simulink model "FrequencyResponseTester"  (R2023b)
settings: Solver=VariableStepAuto  StartTime=0.0  StopTime=10.0  RelTol=1e-3
libraries: simulink x1, c2838x_M4_lib x1
settings Model: Creator=Administrator  LastModifiedBy=Administrator

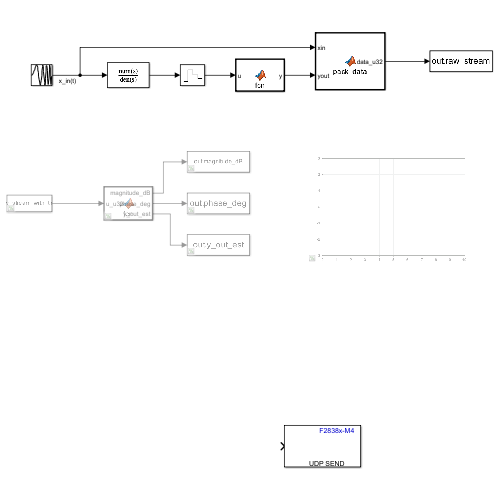
[thumbnail: Simulink's stored preview of the top-level diagram]
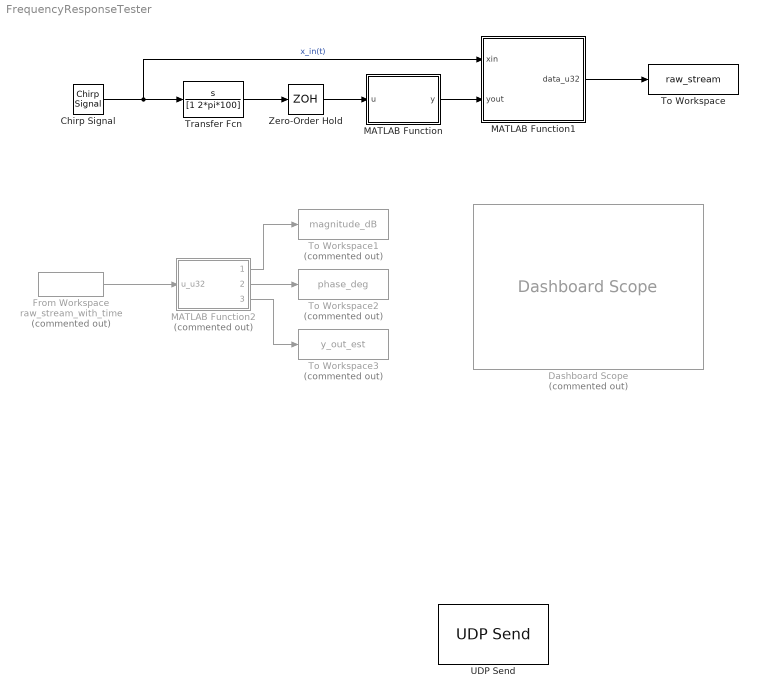
== system FrequencyResponseTester ==
  Chirp Signal : simulink/Sources/Chirp Signal  f1=1  T=10  f2=1000
  Dashboard Scope : DashboardScope  Commented=on
  From Workspace : FromWorkspace  Commented=on  VariableName=raw_stream_with_time  SampleTime=1e-4  OutputAfterFinalValue=Holding final value
  MATLAB Function : MATLAB Function  TreatAsAtomicUnit=on
  MATLAB Function1 : MATLAB Function  TreatAsAtomicUnit=on
  MATLAB Function2 : MATLAB Function  Commented=on  TreatAsAtomicUnit=on
  To Workspace : ToWorkspace  VariableName=raw_stream  SaveFormat=Timeseries  SampleTime=1e-4
  To Workspace1 : ToWorkspace  Commented=on  VariableName=magnitude_dB  SaveFormat=Timeseries  SampleTime=-1
  To Workspace2 : ToWorkspace  Commented=on  VariableName=phase_deg  SaveFormat=Timeseries  SampleTime=-1
  To Workspace3 : ToWorkspace  Commented=on  VariableName=y_out_est  SaveFormat=Timeseries  SampleTime=-1
  Transfer Fcn : TransferFcn  Numerator=[1 0]  Denominator=[1 2*pi*100]
  UDP Send : c2838x_M4_lib/UDP Send  RemoteIPAddress_=127.0.0.1  RemoteIPPort_=25000  LocalIPPort_=-1  BlockingMode=off
  Zero-Order Hold : ZeroOrderHold  SampleTime=1e-4
  wires:
  Chirp Signal/1 -> MATLAB Function1/1(xin), Transfer Fcn/1  "x_in(t)"
  MATLAB Function/1(y) -> MATLAB Function1/2(yout)
  Transfer Fcn/1 -> Zero-Order Hold/1
  Zero-Order Hold/1 -> MATLAB Function/1(u)
  MATLAB Function1/1(data_u32) -> To Workspace/1
  From Workspace/1 -> MATLAB Function2/1(u_u32)
  MATLAB Function2/2(phase_deg) -> To Workspace2/1
  MATLAB Function2/1(magnitude_dB) -> To Workspace1/1
  MATLAB Function2/3(y_out_est) -> To Workspace3/1

== matlab function FrequencyResponseTester/MATLAB Function ==
  data: u input; y output
function y = fcn(u)
    Vref = 10;          % ±5V -> total range 10V
    N = 16;
    q = Vref / 2^N;
    y = round(u / q) * q;
    y = max(-5, min(5, y));  % clamp
end

== matlab function FrequencyResponseTester/MATLAB Function2 ==
  data: u_u32 input; magnitude_dB output; phase_deg output; y_out_est output
function [magnitude_dB, phase_deg, y_out_est] = fcn(u_u32)

% 输入：u_u32 - 来自 From Workspace 的 uint32 数据流
% 输出：
%   magnitude_dB: 幅频响应（dB）
%   phase_deg: 相频响应（度）
%   y_out_est: 预测输出（可选）

coder.extrinsic('process_raw_data');  % 调用外部函数（因为涉及 FFT/Hilbert）

% 调用封装好的处理函数
[mag, phase, yest] = process_raw_data(u_u32);

% 返回输出（注意大小要匹配）
magnitude_dB = mag;
phase_deg = phase;
y_out_est = yest;
assert(length(magnitude_dB) == 4097);
assert(length(phase_deg) == 4097);
assert(length(y_out_est) == 8192);

end

== matlab function FrequencyResponseTester/MATLAB Function1 ==
  data: xin input; data_u32 output; yout input
function data_u32 = pack_data(xin, yout)
% 归一化到 [-1, 1] 并映射到 [0, 65535]

    % 假设输入信号范围是 [-1, 1]，扩展为 [-A, A]
    A = 1;  % 根据实际调整

    % 限制范围
    xin = max(-A, min(A, xin));
    yout = max(-A, min(A, yout));

    % 映射到 [0, 65535]
    x_uint = uint32((xin + A) / (2*A) * 65535);
    y_uint = uint32((yout + A) / (2*A) * 65535);

    % 组合成 uint32: 高16位是 xin, 低16位是 yout
    data_u32 = bitshift(x_uint, 16) + y_uint;
